simulink model "mck3"  (R2021a)
settings: Solver=VariableStepAuto  StartTime=0.0  StopTime=15  MaxStep=0.01  RelTol=1e-3
PreLoadFcn:
  | m=10;
  | c=10;
  | k=30;
settings Model: Creator=seong  LastModifiedBy=pc
settings SolverCC: AlgebraicLoopSolver=TrustRegion
settings DataIOCC: SaveFormat=Array  TimeSaveName=toutmck  OutputSaveName=xdotoutmck
settings DebuggingCC: SFMachineParentedDataDiag=warning
settings SFSimCC: CustomCodeUndefinedFunction=UseInterfaceOnly

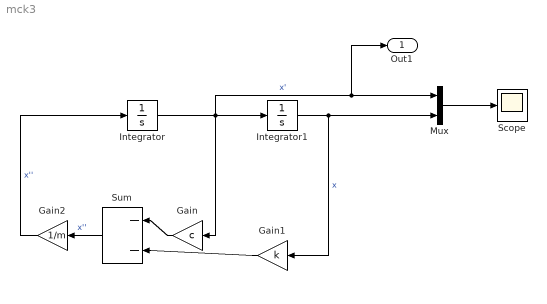
== system mck3 ==
  Gain : Gain  Gain=c
  Gain1 : Gain  Gain=k
  Gain2 : Gain  Gain=1/m
  Integrator : Integrator
  Integrator1 : Integrator  InitialCondition=-5
      settings: AttributesFormatString=x0=-5
  Mux : Mux  Inputs=2
  Scope : Scope
  Sum : Sum  Inputs=|--
  Out1 : Outport
  wires:
  Integrator/1 -> Out1/1, Mux/1, Gain/1, Integrator1/1  "x'"
  Gain2/1 -> Integrator/1  "x''"
  Integrator1/1 -> Mux/2, Gain1/1  "x"
  Gain1/1 -> Sum/2
  Gain/1 -> Sum/1
  Sum/1 -> Gain2/1  "x''"
  Mux/1 -> Scope/1
